simulink model "Ques7Ex2_AkankshaMurali"  (R2023b)
settings: Solver=VariableStepAuto  StartTime=0.0  StopTime=10.0  RelTol=1e-3
settings Model: Creator=akank  LastModifiedBy=akank

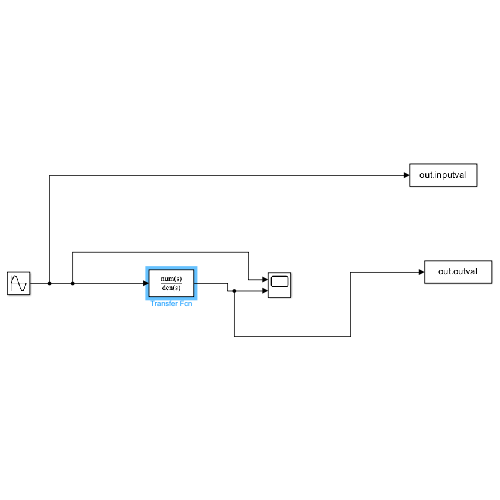
[thumbnail: Simulink's stored preview of the top-level diagram]
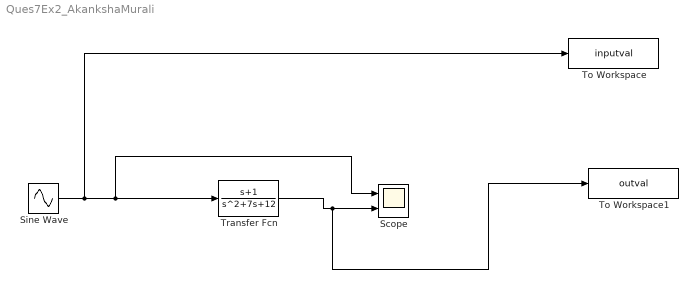
== system Ques7Ex2_AkankshaMurali ==
  Scope : Scope  NumInputPorts=2
  Sine Wave : Sin  Amplitude=1.79  Frequency=31.4159265  SampleTime=0
  To Workspace : ToWorkspace  VariableName=inputval  SaveFormat=Timeseries  SampleTime=-1
  To Workspace1 : ToWorkspace  VariableName=outval  SaveFormat=Timeseries  SampleTime=-1
  Transfer Fcn : TransferFcn  Numerator=[1 1]  Denominator=[1 7 12]
  wires:
  Sine Wave/1 -> To Workspace/1, Scope/1, Transfer Fcn/1
  Transfer Fcn/1 -> To Workspace1/1, Scope/2
